simulink model "Q3sim6"  (R2022a)
settings: Solver=VariableStepAuto  StartTime=0.0  StopTime=30  FixedStep=1e-4  RelTol=1e-3
values from neighbouring files (symbols this model uses):
  A = [zeros(4,1) A]    [Q3.m]
  Am = M    (= 0)    [Q3.m]
  B = B(:,1)    [Q3.m]
  Bm = N    (= 1)    [Q3.m]
  C = [1 0 0 0]    [Q3.m]
  K = Ka (1:4)    [Q3.m]
  Km = Ka(5)    [Q3.m]
  L = lqr(A',C',Ql,Rl)'    [Q3.m]
  x0obs = [0 0 0 0]    [Q3.m]
settings Model: Creator=Crippa  LastModifiedBy=Crippa
settings SolverCC: ZeroCrossControl=DisableAll

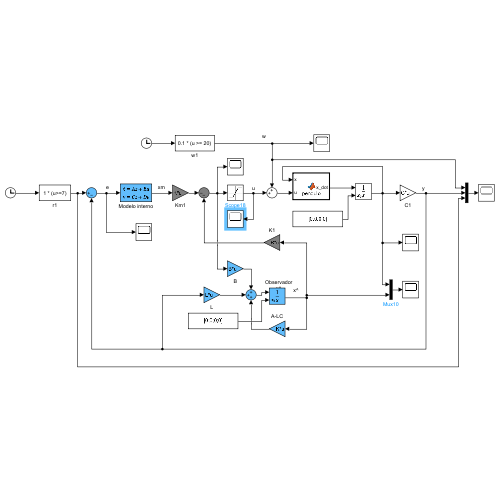
[thumbnail: Simulink's stored preview of the top-level diagram]
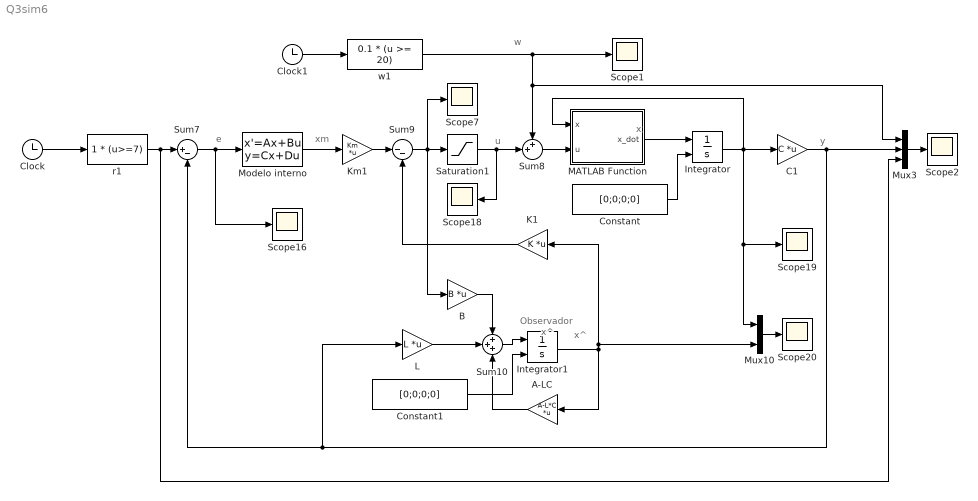
== system Q3sim6 ==
  note: w
  note: u
  note: x
  note: xm
  note: Observador
  note: x^
  note: e
  note: y
  note: x^
  A-LC : Gain  Gain=A-L*C  Multiplication=Matrix(K*u)
  B : Gain  Gain=B  Multiplication=Matrix(K*u)
  C1 : Gain  Gain=C  Multiplication=Matrix(K*u)
  Clock : Clock
  Clock1 : Clock
  Constant : Constant  Value=[0;0;0;0]  VectorParams1D=off
  Constant1 : Constant  Value=[0;0;0;0]  VectorParams1D=off
  Integrator : Integrator  InitialConditionSource=external
  Integrator1 : Integrator  InitialConditionSource=external  InitialCondition=x0obs
  K1 : Gain  Gain=K  Multiplication=Matrix(K*u)
  Km1 : Gain  Gain=Km  Multiplication=Matrix(K*u)
  L : Gain  Gain=L  Multiplication=Matrix(K*u)
  MATLAB Function : MATLAB Function  TreatAsAtomicUnit=on
  Modelo interno : StateSpace  A=Am  B=Bm  C=eye(1)  D=zeros(1)  InitialCondition=0
  Mux10 : Mux  Inputs=2
  Mux3 : Mux  Inputs=3
  Saturation1 : Saturate  UpperLimit=150  LowerLimit=-150
  Scope{1..2,7,16,18..20} (7 alike) : Scope
  Sum10 : Sum  Inputs=+++
  Sum7 : Sum  Inputs=|+-
  Sum8 : Sum  Inputs=++|
  Sum9 : Sum  Inputs=|--
  r1 : Fcn  Expr=1 * (u>=7)
  w1 : Fcn  Expr=0.1 * (u >= 20)
  wires:
  Mux3/1 -> Scope2/1
  Clock1/1 -> w1/1
  w1/1 -> Scope1/1, Sum8/1, Mux3/1
  Sum10/1 -> Integrator1/1
  Mux10/1 -> Scope20/1
  K1/1 -> Sum9/2
  Integrator1/1 -> Mux10/2, K1/1, A-LC/1
  C1/1 -> Mux3/2, L/1, Sum7/2
  B/1 -> Sum10/1
  A-LC/1 -> Sum10/3
  Sum7/1 -> Modelo interno/1, Scope16/1
  Km1/1 -> Sum9/1
  Saturation1/1 -> Sum8/2, Scope18/1
  r1/1 -> Mux3/3, Sum7/1
  Sum9/1 -> Scope7/1, B/1, Saturation1/1
  L/1 -> Sum10/2
  Modelo interno/1 -> Km1/1
  Sum8/1 -> MATLAB Function/2(u)
  Clock/1 -> r1/1
  Constant/1 -> Integrator/2
  MATLAB Function/1(x_dot) -> Integrator/1
  Integrator/1 -> MATLAB Function/1(x), Mux10/1, Scope19/1, C1/1
  Constant1/1 -> Integrator1/2

== matlab function Q3sim6/MATLAB Function ==
  data: x input; u input; x_dot output
function x_dot = pendulo(x,u)
    % x1 = y, x2 = y', x3 = theta, x4 = theta'

    % Parâmetros do pêndulo invertido
    M = 1; 
    m = 0.5;
    L = 1; 
    g = 9.81;

    x1 = x(1);
    x2 = x(2);
    x3 = x(3);
    x4 = x(4);

    % Dinâmica dos estados
    f1 = x2;
    f2 = (-m*g*sin(x3)*cos(x3) + m*L*(x4^2)*sin(x3)) / (M+m-m*cos(x3)^2);
    f3 = x4;
    f4 = g*sin(x3)/L - f2*cos(x3)/L;
    
    % Dinâmica do controle
    g1 = 0;
    g2 = u/(M+m-m*cos(x3)^2);
    g3 = 0;
    g4 = -cos(x3)/L * u/(M+m-m*cos(x3)^2);
    
    f = [f1; f2; f3; f4];
    g = [g1; g2; g3; g4];

    x_dot = f + g;
end
